simulink model "Observer_bandwidth"  (R2021b)
settings: Solver=VariableStepAuto  StartTime=0.0  StopTime=30  RelTol=1e-3
values from neighbouring files (symbols this model uses):
  F_mimo = -place(A,B,Desired_poles)    [SS_MIMO.m]    (also in controller_code.m = [-2457.0,      0,      0,       0, -193.7,      0,      0,  )
  L_mimo = -place(A',C',Desired_poles_obs)'    [SS_MIMO.m]
  sys_mimo = ss(A,B,C,0)    [SS_MIMO.m]
libraries: simulink_extras x4
settings Model: Creator=krist  LastModifiedBy=krist
settings SolverCC: AlgebraicLoopSolver=TrustRegion
settings DebuggingCC: SFMachineParentedDataDiag=warning

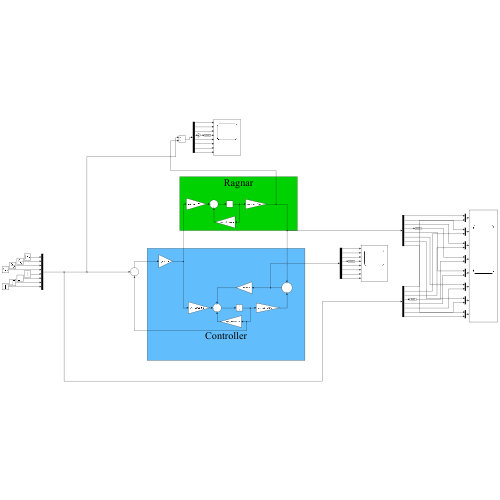
[thumbnail: Simulink's stored preview of the top-level diagram]
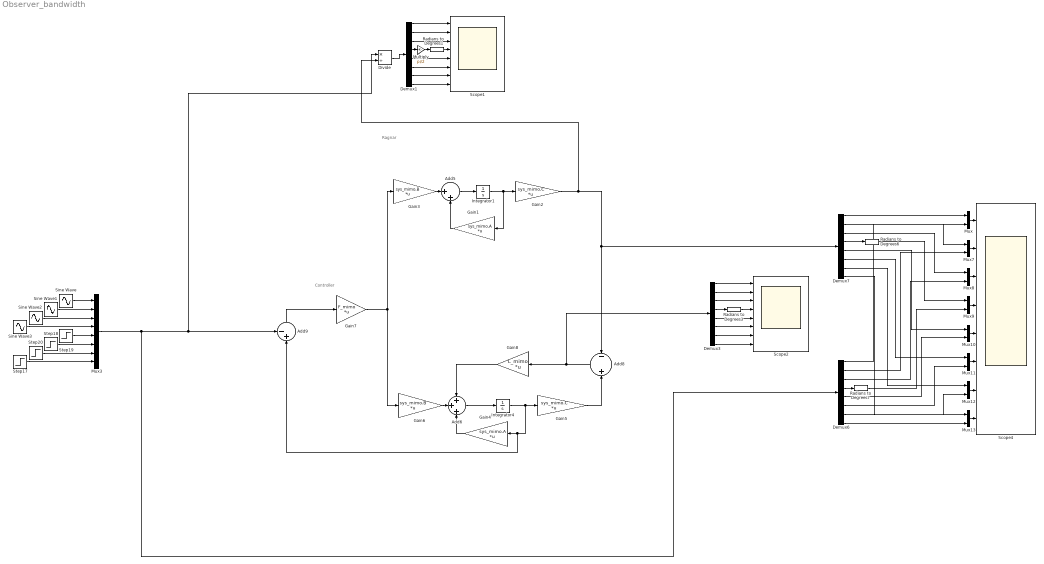
== system Observer_bandwidth ==
  note: Ragnar
  note: Controller
  Add5 : Sum  Inputs=|++
  Add6 : Sum  Inputs=+++
  Add8 : Sum  Inputs=-+
  Add9 : Sum  Inputs=-+|
  Demux{1,3,6..7} (4 alike) : Demux  Outputs=8
  Divide : Product  Inputs=*/
  Gain1 : Gain  Gain=sys_mimo.A  Multiplication=Matrix(K*u)
  Gain2 : Gain  Gain=sys_mimo.C  Multiplication=Matrix(K*u)
  Gain3 : Gain  Gain=sys_mimo.B  Multiplication=Matrix(K*u)
  Gain4 : Gain  Gain=sys_mimo.A  Multiplication=Matrix(K*u)
  Gain5 : Gain  Gain=sys_mimo.C  Multiplication=Matrix(K*u)
  Gain6 : Gain  Gain=sys_mimo.B  Multiplication=Matrix(K*u)
  Gain7 : Gain  Gain=F_mimo  Multiplication=Matrix(K*u)
  Gain8 : Gain  Gain=L_mimo  Multiplication=Matrix(K*u)
  Integrator1 : Integrator  InitialCondition=[0 0.5 -0.4 deg2rad(90) 0 0 0 0]
  Integrator4 : Integrator  InitialCondition=[0 0.55 -0.35 deg2rad(93) 0 0 0 0]
  Multiply : Gain  Gain=pi/2
  Mux{,7..13} (8 alike) : Mux  Inputs=2
  Mux3 : Mux  Inputs=8
  Radians to Degrees{1,3,6..7} (4 alike) : simulink_extras/Transformations/Radians to Degrees
  Scope1 : Scope  NumInputPorts=8
  Scope2 : Scope  NumInputPorts=8
  Scope4 : Scope  NumInputPorts=8
  Sine Wave : Sin  Amplitude=0.01  Frequency=0.5  SampleTime=0
  Sine Wave1 : Sin  Amplitude=0.01  Bias=0.5  Frequency=0.5  SampleTime=0
  Sine Wave2 : Sin  Amplitude=0.01  Bias=-0.4  Frequency=0.5  SampleTime=0
  Sine Wave3 : Sin  Amplitude=deg2rad(5)  Bias=deg2rad(90)  Frequency=0.5  SampleTime=0
  Step{17..20} (4 alike) : Step  Time=0  After=0  SampleTime=1
  wires:
  Add8/1 -> Demux3/1, Gain8/1
  Gain1/1 -> Add5/2
  Integrator1/1 -> Gain1/1, Gain2/1
  Add5/1 -> Integrator1/1
  Gain3/1 -> Add5/1
  Mux3/1 -> Demux6/1, Divide/1, Add9/1
  Add6/1 -> Integrator4/1
  Gain4/1 -> Add6/3
  Gain8/1 -> Add6/1
  Gain6/1 -> Add6/2
  Sine Wave3/1 -> Mux3/4
  Sine Wave2/1 -> Mux3/3
  Sine Wave/1 -> Mux3/1
  Sine Wave1/1 -> Mux3/2
  Step18/1 -> Mux3/6
  Step17/1 -> Mux3/8
  Step20/1 -> Mux3/7
  Step19/1 -> Mux3/5
  Integrator4/1 -> Add9/2, Gain4/1, Gain5/1
  Gain5/1 -> Add8/2
  Demux7/8 -> Mux13/1
  Demux7/3 -> Mux8/1
  Demux7/2 -> Mux7/1
  Gain2/1 -> Divide/2, Add8/1, Demux7/1
  Demux7/1 -> Mux/1
  Demux7/4 -> Radians to Degrees6/1
  Demux6/4 -> Radians to Degrees7/1
  Mux/1 -> Scope4/1
  Mux7/1 -> Scope4/2
  Mux8/1 -> Scope4/3
  Mux9/1 -> Scope4/4
  Mux13/1 -> Scope4/8
  Mux12/1 -> Scope4/7
  Mux10/1 -> Scope4/5
  Mux11/1 -> Scope4/6
  Radians to Degrees6/1 -> Mux9/1
  Demux7/5 -> Mux10/1
  Demux7/6 -> Mux11/1
  Demux7/7 -> Mux12/1
  Demux6/8 -> Mux13/2
  Demux6/7 -> Mux12/2
  Demux6/6 -> Mux11/2
  Demux6/5 -> Mux10/2
  Radians to Degrees7/1 -> Mux9/2
  Demux6/3 -> Mux8/2
  Demux6/2 -> Mux7/2
  Demux6/1 -> Mux/2
  Demux3/6 -> Scope2/6
  Demux3/7 -> Scope2/7
  Demux3/1 -> Scope2/1
  Demux3/2 -> Scope2/2
  Demux3/4 -> Radians to Degrees3/1
  Radians to Degrees3/1 -> Scope2/4
  Demux3/8 -> Scope2/8
  Demux3/3 -> Scope2/3
  Demux3/5 -> Scope2/5
  Add9/1 -> Gain7/1
  Gain7/1 -> Gain6/1, Gain3/1
  Demux1/7 -> Scope1/7
  Demux1/5 -> Scope1/5
  Demux1/6 -> Scope1/6
  Demux1/8 -> Scope1/8
  Demux1/3 -> Scope1/3
  Demux1/2 -> Scope1/2
  Demux1/1 -> Scope1/1
  Divide/1 -> Demux1/1
  Radians to Degrees1/1 -> Scope1/4
  Demux1/4 -> Multiply/1
  Multiply/1 -> Radians to Degrees1/1
